simulink model "test_IdInput_Block"  (Simulink 4.00)
settings: Solver=FixedStepDiscrete  StartTime=0.0  StopTime=100  FixedStep=0.05  RelTol=1e-3
values from neighbouring files (symbols this model uses):
  prbs_data = [10.05 10.1 10.15 10.2 10.25 10.3 10.35 10.4 10.45 10.5 10.55 10.6 ... (3200 elements, 1600x2)]    [prbs_data.mat]
libraries: IdInput_block_lib x1
settings Model: LastModifiedBy=bsaunder

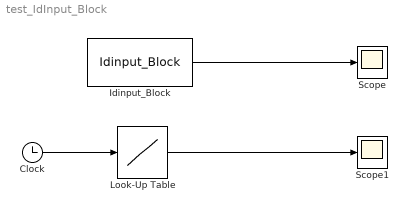
== system test_IdInput_Block ==
  Clock : Clock
      settings: DisplayTime=off  Decimation=10
  Idinput_Block : IdInput_block_lib/Idinput_Block  ssT=[10 30]  signal_type=PRBS  band=[0 1/16]  levels=[3.2 3.8]  Ts=0.05
  Look-Up Table : Lookup  InputValues=[0 prbs_data(:,1)' prbs_data(end,1)+0.05 prbs_data(end,1)+0.10]  OutputValues=[0 ((400-300).*prbs_data(:,2)')+300 0 0]
  Scope : Scope
      settings: TimeRange=auto  YMin=-5  YMax=5  SaveToWorkspace=off  SaveName=ScopeData  LimitDataPoints=on  MaxDataPoints=5000
  Scope1 : Scope
      settings: TimeRange=auto  YMin=-5  YMax=5  SaveToWorkspace=off  LimitDataPoints=on  MaxDataPoints=5000
  wires:
  Idinput_Block/1 -> Scope/1
  Look-Up Table/1 -> Scope1/1
  Clock/1 -> Look-Up Table/1
